simulink subsystem "sensor_model"  (R2023a)
settings: Solver=VariableStepAuto  StartTime=0.0  StopTime=10.0  RelTol=1e-3
undefined symbols (not defined in the file): Earth, latitude, longitude, param, WGS84
libraries: dspfdesign x6, simulink_extras x3, aerolibatmos2 x2, sensorgpslib x1, aerolibtransform2 x1, aerolibnav x1
settings Model: Creator=timme  LastModifiedBy=timme

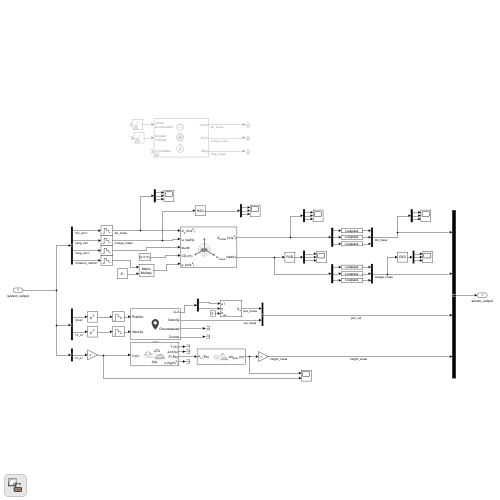
[thumbnail: Simulink's stored preview of the top-level diagram]
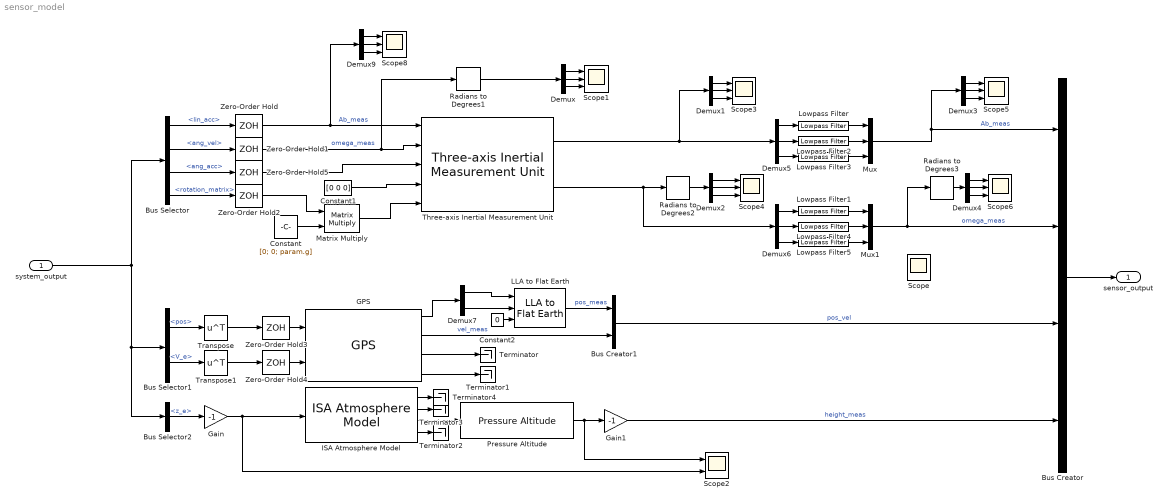
== system sensor_model ==
  system_output : Inport
  Bus Creator : BusCreator  Inputs=4
  Bus Creator1 : BusCreator  Inputs=2
  Bus Selector : BusSelector  OutputSignals=lin_acc,ang_vel,ang_acc,rotation_matrix
  Bus Selector1 : BusSelector  OutputSignals=pos,V_e
  Bus Selector2 : BusSelector  OutputSignals=pos.z_e
  Constant : Constant  Value=[0; 0; param.g]
  Constant1 : Constant  Value=[0 0 0]
  Constant2 : Constant  Value=0
  Demux{,1..6,9} (8 alike) : Demux  Outputs=3
  Demux7 : Demux  Outputs=[2 1]
  GPS : sensorgpslib/GPS  DispRefFrame=NED  PositionInputFormat=Local  ReferenceLocation=[latitude, longitude, 0]  HorizontalPositionAccuracy=1.6  VerticalPositionAccuracy=3  VelocityAccuracy=0.1  DecayFactor=0.999  SeedDouble=67  SimulateUsing=Interpreted execution
      settings: LibrarySourceBlock=uavsimlib/GPS
  Gain : Gain  Gain=-1
  Gain1 : Gain  Gain=-1
  ISA Atmosphere Model : aerolibatmos2/ISA Atmosphere Model  custom=off  g=9.80665  gamma=1.4  R=287.0531  L=0.0065  h_trop=11000  h_strat=20000  rho0=1.225  P0=101325  T0=288.15  h0=0
  LLA to Flat Earth : aerolibtransform2/LLA to Flat Earth  units=Metric (MKS)  ptype=Earth (WGS84)  F=1/298.257223563  R=6378137  refPosPort=off  LL0=[latitude longitude]  psi=0
  Lowpass Filter : dspfdesign/Lowpass Filter  FilterType=IIR  DesignForMinimumOrder=on  FilterOrder=50  PassbandFrequency=50  StopbandFrequency=499  PassbandRipple=0.1  StopbandAttenuation=80  SampleRateMode=Specify on dialog  SampleRate=1000  SimulateUsing=Interpreted execution  roundingMode=Floor  coeffsDataTypeStr=fixdt(1,16)
  Lowpass Filter1 : dspfdesign/Lowpass Filter  FilterType=IIR  DesignForMinimumOrder=on  FilterOrder=50  PassbandFrequency=25  StopbandFrequency=499  PassbandRipple=0.1  StopbandAttenuation=80  SampleRateMode=Specify on dialog  SampleRate=1000  SimulateUsing=Interpreted execution  roundingMode=Floor  coeffsDataTypeStr=fixdt(1,16)
  Lowpass Filter2 : dspfdesign/Lowpass Filter  FilterType=IIR  DesignForMinimumOrder=on  FilterOrder=50  PassbandFrequency=50  StopbandFrequency=499  PassbandRipple=0.1  StopbandAttenuation=80  SampleRateMode=Specify on dialog  SampleRate=1000  SimulateUsing=Interpreted execution  roundingMode=Floor  coeffsDataTypeStr=fixdt(1,16)
  Lowpass Filter3 : dspfdesign/Lowpass Filter  FilterType=IIR  DesignForMinimumOrder=on  FilterOrder=50  PassbandFrequency=50  StopbandFrequency=499  PassbandRipple=0.1  StopbandAttenuation=80  SampleRateMode=Specify on dialog  SampleRate=1000  SimulateUsing=Interpreted execution  roundingMode=Floor  coeffsDataTypeStr=fixdt(1,16)
  Lowpass Filter4 : dspfdesign/Lowpass Filter  FilterType=IIR  DesignForMinimumOrder=on  FilterOrder=50  PassbandFrequency=25  StopbandFrequency=499  PassbandRipple=0.1  StopbandAttenuation=80  SampleRateMode=Specify on dialog  SampleRate=1000  SimulateUsing=Interpreted execution  roundingMode=Floor  coeffsDataTypeStr=fixdt(1,16)
  Lowpass Filter5 : dspfdesign/Lowpass Filter  FilterType=IIR  DesignForMinimumOrder=on  FilterOrder=50  PassbandFrequency=25  StopbandFrequency=499  PassbandRipple=0.1  StopbandAttenuation=80  SampleRateMode=Specify on dialog  SampleRate=1000  SimulateUsing=Interpreted execution  roundingMode=Floor  coeffsDataTypeStr=fixdt(1,16)
  Matrix Multiply : Product  Multiplication=Matrix(*)
  Mux : Mux  Inputs=3
  Mux1 : Mux  Inputs=3
  Pressure Altitude : aerolibatmos2/Pressure Altitude  units=Metric (MKS)  action=Warning
  Radians to Degrees1 : simulink_extras/Transformations/Radians to Degrees
  Radians to Degrees2 : simulink_extras/Transformations/Radians to Degrees
  Radians to Degrees3 : simulink_extras/Transformations/Radians to Degrees
  Scope : Scope  NumInputPorts=2
  Scope{1,3..6,8} (6 alike) : Scope  NumInputPorts=3
  Scope2 : Scope  NumInputPorts=2
  Terminator{,1..4} (5 alike) : Terminator
  Three-axis Inertial Measurement Unit : aerolibnav/Three-axis Inertial Measurement Unit  units=Metric (MKS)  imu=[0 0 0]  i_Ts=0.001  dtype_a=on  w_a=190  z_a=0.707  a_sf_cc=[1 0 0; 0 1 0; 0 0 1]  a_bias=[0 0 0]  a_sat="[-inf  -inf  -inf  inf inf inf]"  dtype_g=on  w_g=190  z_g=0.707  g_sf_cc=[1 0 0; 0 1 0; 0 0 1]  g_bias=[0 0 0]  g_sens=[0 0 0]  g_sat="[-inf  -inf  -inf  inf inf inf]"  i_rand=on  i_seeds=[23093 23094 23095 23096 23097 23098]  i_pow=[0.0001 0.0001 0.0001 0.00001 0.00001 0.00001]
  Transpose : Math  Operator=transpose
  Transpose1 : Math  Operator=transpose
  Zero-Order Hold{,1..2,5} (4 alike) : ZeroOrderHold  SampleTime=0.001
  Zero-Order Hold3 : ZeroOrderHold  SampleTime=0.1
  Zero-Order Hold4 : ZeroOrderHold  SampleTime=0.1
  sensor_output : Outport
  wires:
  LLA to Flat Earth/1 -> Bus Creator1/1  "pos_meas"
  Gain1/1 -> Bus Creator/4  "height_meas"
  GPS/2 -> Bus Creator1/2  "vel_meas"
  Bus Creator1/1 -> Bus Creator/3  "pos_vel"
  Transpose/1 -> Zero-Order Hold3/1
  Demux7/2 -> LLA to Flat Earth/2
  Zero-Order Hold1/1 -> Three-axis Inertial Measurement Unit/2, Radians to Degrees1/1  "omega_meas"
  ISA Atmosphere Model/1 -> Terminator4/1
  Bus Selector/4 -> Zero-Order Hold2/1  "<rotation_matrix>"
  Gain/1 -> ISA Atmosphere Model/1, Scope2/2
  GPS/3 -> Terminator/1
  GPS/4 -> Terminator1/1
  Bus Selector1/1 -> Transpose/1  "<pos>"
  ISA Atmosphere Model/3 -> Pressure Altitude/1
  Pressure Altitude/1 -> Gain1/1, Scope2/1
  Bus Selector2/1 -> Gain/1  "<z_e>"
  Bus Selector/2 -> Zero-Order Hold1/1  "<ang_vel>"
  Bus Selector/1 -> Zero-Order Hold/1  "<lin_acc>"
  ISA Atmosphere Model/4 -> Terminator2/1
  Transpose1/1 -> Zero-Order Hold4/1
  Zero-Order Hold3/1 -> GPS/1
  Zero-Order Hold4/1 -> GPS/2
  GPS/1 -> Demux7/1
  Constant2/1 -> LLA to Flat Earth/3
  Bus Selector1/2 -> Transpose1/1  "<V_e>"
  Demux7/1 -> LLA to Flat Earth/1
  ISA Atmosphere Model/2 -> Terminator3/1
  Bus Creator/1 -> sensor_output/1
  Demux/2 -> Scope1/2
  Demux/1 -> Scope1/1
  Demux/3 -> Scope1/3
  Zero-Order Hold2/1 -> Matrix Multiply/1
  Demux1/2 -> Scope3/2
  Demux1/3 -> Scope3/3
  Demux1/1 -> Scope3/1
  Radians to Degrees1/1 -> Demux/1
  Bus Selector/3 -> Zero-Order Hold5/1  "<ang_acc>"
  Constant/1 -> Matrix Multiply/2
  Radians to Degrees2/1 -> Demux2/1
  Demux2/3 -> Scope4/3
  Demux2/1 -> Scope4/1
  Demux2/2 -> Scope4/2
  Three-axis Inertial Measurement Unit/1 -> Demux5/1, Demux1/1
  Three-axis Inertial Measurement Unit/2 -> Radians to Degrees2/1, Demux6/1
  Zero-Order Hold/1 -> Three-axis Inertial Measurement Unit/1, Demux9/1  "Ab_meas"
  Zero-Order Hold5/1 -> Three-axis Inertial Measurement Unit/3
  Constant1/1 -> Three-axis Inertial Measurement Unit/4
  Matrix Multiply/1 -> Three-axis Inertial Measurement Unit/5
  Demux3/3 -> Scope5/3
  Demux3/2 -> Scope5/2
  Demux3/1 -> Scope5/1
  Demux4/1 -> Scope6/1
  Demux4/2 -> Scope6/2
  Demux4/3 -> Scope6/3
  Mux1/1 -> Bus Creator/2, Radians to Degrees3/1  "omega_meas"
  Radians to Degrees3/1 -> Demux4/1
  Demux5/1 -> Lowpass Filter/1
  Lowpass Filter/1 -> Mux/1
  Demux5/2 -> Lowpass Filter2/1
  Lowpass Filter2/1 -> Mux/2
  Demux5/3 -> Lowpass Filter3/1
  Lowpass Filter3/1 -> Mux/3
  Demux6/1 -> Lowpass Filter1/1
  Demux6/3 -> Lowpass Filter5/1
  Lowpass Filter5/1 -> Mux1/3
  Lowpass Filter1/1 -> Mux1/1
  Lowpass Filter4/1 -> Mux1/2
  Demux6/2 -> Lowpass Filter4/1
  Demux9/3 -> Scope8/3
  Demux9/2 -> Scope8/2
  Demux9/1 -> Scope8/1
  system_output/1 -> Bus Selector2/1, Bus Selector1/1, Bus Selector/1
  Mux/1 -> Demux3/1, Bus Creator/1  "Ab_meas"
